simulink model "two_area_model"  (R2016b)
settings: Solver=VariableStepAuto  StartTime=0.0  StopTime=10.0  RelTol=1e-3
values from neighbouring files (symbols this model uses):
  B_freq = 1/S    (= 25)    [run_simulation.m]
  C_p = 0.17    [run_simulation.m]
  D_L = 1/200    (= 0.005)    [run_simulation.m]
  J = [J11 J12(:,idx_pq) J13; J21(idx_pq,:) J22(idx_pq,idx_pq) J23(idx_pq)]    [pf_with_AGC.m]    (also in run_simulation.m = 40)
  P_hat = 1/S    (= 25)    [run_simulation.m]
  S = 0.04    [run_simulation.m]
  T_N = 120    [run_simulation.m]
  T_t = 0    [run_simulation.m]
  w0 = 50    [run_simulation.m]
  W_0 = 0    [run_simulation.m]
settings Model: Creator=dc  LastModifiedBy=dc

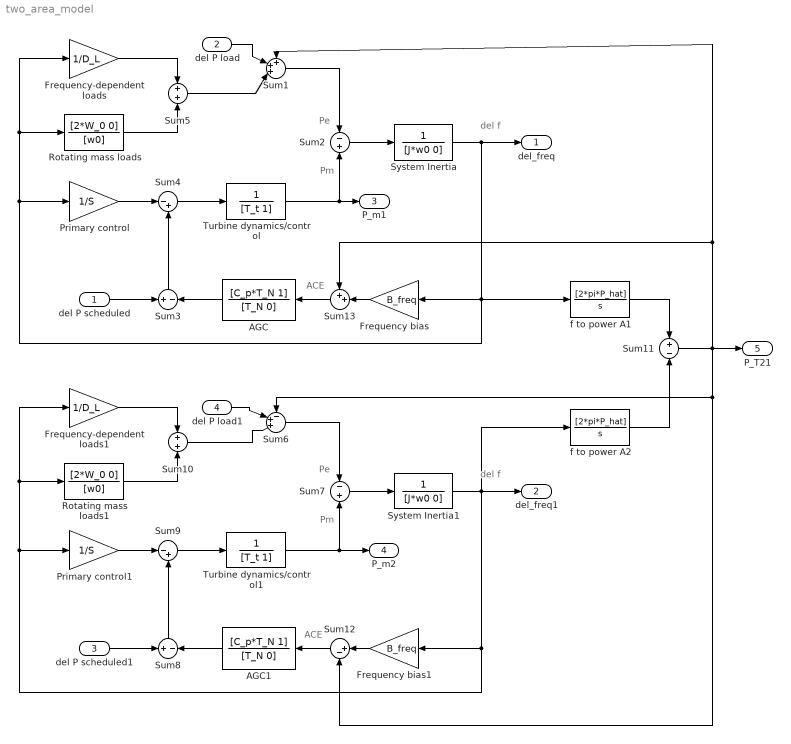
== system two_area_model ==
  note: Pm
  note: Pe
  note: ACE
  note: del f
  note: Pm
  note: Pe
  note: ACE
  note: del f
  del P scheduled : Inport
  del P load : Inport  Port=2
  del P scheduled1 : Inport  Port=3
  del P load1 : Inport  Port=4
  AGC : TransferFcn  Numerator=[C_p*T_N 1]  Denominator=[T_N 0]
  AGC1 : TransferFcn  Numerator=[C_p*T_N 1]  Denominator=[T_N 0]
  Frequency bias : Gain  Gain=B_freq
  Frequency bias1 : Gain  Gain=B_freq
  Frequency-dependent loads : Gain  Gain=1/D_L
  Frequency-dependent loads1 : Gain  Gain=1/D_L
  Primary control : Gain  Gain=1/S
  Primary control1 : Gain  Gain=1/S
  Rotating mass loads : TransferFcn  Numerator=[2*W_0 0]  Denominator=[w0]
  Rotating mass loads1 : TransferFcn  Numerator=[2*W_0 0]  Denominator=[w0]
  Sum1 : Sum  Inputs=+++|
  Sum10 : Sum  Inputs=+|+
  Sum11 : Sum  Inputs=+|-
  Sum12 : Sum  Inputs=|+-
  Sum13 : Sum  Inputs=++|
  Sum2 : Sum  Inputs=-|+
  Sum3 : Sum  Inputs=+|-
  Sum4 : Sum  Inputs=|-+
  Sum5 : Sum  Inputs=+|+
  Sum6 : Sum  Inputs=-++|
  Sum7 : Sum  Inputs=-|+
  Sum8 : Sum  Inputs=+|-
  Sum9 : Sum  Inputs=|-+
  System Inertia : TransferFcn  Denominator=[J*w0 0]
  System Inertia1 : TransferFcn  Denominator=[J*w0 0]
  Turbine dynamics/control : TransferFcn  Denominator=[T_t 1]
  Turbine dynamics/control1 : TransferFcn  Denominator=[T_t 1]
  f to power A1 : TransferFcn  Numerator=[2*pi*P_hat]  Denominator=[1 0]
  f to power A2 : TransferFcn  Numerator=[2*pi*P_hat]  Denominator=[1 0]
  del_freq : Outport
  del_freq1 : Outport  Port=2
  P_m1 : Outport  Port=3
  P_m2 : Outport  Port=4
  P_T21 : Outport  Port=5
  wires:
  Frequency-dependent loads/1 -> Sum5/1
  Rotating mass loads/1 -> Sum5/2
  Sum2/1 -> System Inertia/1
  Turbine dynamics/control/1 -> P_m1/1, Sum2/2
  Sum1/1 -> Sum2/1
  System Inertia/1 -> del_freq/1, f to power A1/1, Rotating mass loads/1, Frequency-dependent loads/1, Primary control/1, Frequency bias/1
  Frequency bias/1 -> Sum13/2
  Sum4/1 -> Turbine dynamics/control/1
  Primary control/1 -> Sum4/1
  Sum3/1 -> Sum4/2
  AGC/1 -> Sum3/2
  Sum5/1 -> Sum1/3
  del P load/1 -> Sum1/2
  del P scheduled/1 -> Sum3/1
  Frequency-dependent loads1/1 -> Sum10/1
  Rotating mass loads1/1 -> Sum10/2
  Sum7/1 -> System Inertia1/1
  Turbine dynamics/control1/1 -> P_m2/1, Sum7/2
  Sum6/1 -> Sum7/1
  System Inertia1/1 -> f to power A2/1, del_freq1/1, Rotating mass loads1/1, Frequency-dependent loads1/1, Primary control1/1, Frequency bias1/1
  Frequency bias1/1 -> Sum12/1
  Sum9/1 -> Turbine dynamics/control1/1
  Primary control1/1 -> Sum9/1
  Sum8/1 -> Sum9/2
  AGC1/1 -> Sum8/2
  Sum10/1 -> Sum6/3
  del P load1/1 -> Sum6/2
  del P scheduled1/1 -> Sum8/1
  f to power A1/1 -> Sum11/1
  f to power A2/1 -> Sum11/2
  Sum12/1 -> AGC1/1
  Sum13/1 -> AGC/1
  Sum11/1 -> P_T21/1, Sum6/1, Sum12/2, Sum13/1, Sum1/1
